simulink model "GolfSwing"  (R2024b)
settings: Solver=VariableStepAuto  StartTime=0.0  StopTime=StopTime  MaxStep=0.001  RelTol=1e-3
PreLoadFcn:
  | cd(matlabdrive);
  | cd '2DModel';
PostLoadFcn:
  | %run SCRIPT_mdlWksGenerate.m;
  | mdlWks=get_param('GolfSwing','ModelWorkspace');
  | mdlWks.DataSource = 'MAT-File';
  | mdlWks.FileName = 'ModelInputs.mat';
  | mdlWks.reload;
model workspace: external: MAT-File ModelInputs.mat (data not in the file)
undefined symbols (not defined in the file or in its folder): GlobalGain, HipConstant, HipDampening, HipTimeGain, KillDampFinalValue, KillDampInitialValue, KillswitchFinalValue, KillswitchInitialValue, KillswitchStepTime, LElbowConstant, LElbowDampening, LElbowTimeGain, LScapConstant, LScapDampening, LScapPositionGain, LScapTimeGain, LShoulderConstant, LShoulderDampening, LShoulderTimeGain, LWristConstant, LWristDampening, LWristTimeGain, RElbowConstant, RElbowDampening, RElbowTimeGain, RScapConstant, RScapDampening, RScapPositionGain, RScapTimeGain, RShoulderConstant, RShoulderDampening, RShoulderTimeGain, RWristConstant, RWristDampening, RWristTimeGain, TorsoConstant, TorsoDampening, TorsoPositionGain, TorsoTimeGain, WristGain, X, Y, Z
libraries: nesl_utility x207, sm_lib x106, matrix_library x11, simulink_extras x2, simulink x1
(part 6 of 6)

== system GolfSwing/Club/RWGlobal ==
  Add : Sum  Inputs=+++
  Math Function : Math  Operator=square
  Math Function1 : Math  Operator=square
  Math Function2 : Math  Operator=square
  Mux : Mux  Inputs=3
  Mux1 : Mux  Inputs=3
  RWAV : nesl_utility/PS-Simulink Converter  PhysicalDomain=network_engine_domain  SubClassName=ps_output  LeftPortType=input  RightPortType=output  PseudoPeriodic=off  Frequencies=[]  VectorFormat=1-D array  Unit=inherit  AffineConversion=off
  RWvx : nesl_utility/PS-Simulink Converter  PhysicalDomain=network_engine_domain  SubClassName=ps_output  LeftPortType=input  RightPortType=output  PseudoPeriodic=off  Frequencies=[]  VectorFormat=1-D array  Unit=inherit  AffineConversion=off
  RWvy : nesl_utility/PS-Simulink Converter  PhysicalDomain=network_engine_domain  SubClassName=ps_output  LeftPortType=input  RightPortType=output  PseudoPeriodic=off  Frequencies=[]  VectorFormat=1-D array  Unit=inherit  AffineConversion=off
  RWvz : nesl_utility/PS-Simulink Converter  PhysicalDomain=network_engine_domain  SubClassName=ps_output  LeftPortType=input  RightPortType=output  PseudoPeriodic=off  Frequencies=[]  VectorFormat=1-D array  Unit=inherit  AffineConversion=off
  RWx : nesl_utility/PS-Simulink Converter  PhysicalDomain=network_engine_domain  SubClassName=ps_output  LeftPortType=input  RightPortType=output  PseudoPeriodic=off  Frequencies=[]  VectorFormat=1-D array  Unit=inherit  AffineConversion=off
  RWy : nesl_utility/PS-Simulink Converter  PhysicalDomain=network_engine_domain  SubClassName=ps_output  LeftPortType=input  RightPortType=output  PseudoPeriodic=off  Frequencies=[]  VectorFormat=1-D array  Unit=inherit  AffineConversion=off
  RWz : nesl_utility/PS-Simulink Converter  PhysicalDomain=network_engine_domain  SubClassName=ps_output  LeftPortType=input  RightPortType=output  PseudoPeriodic=off  Frequencies=[]  VectorFormat=1-D array  Unit=inherit  AffineConversion=off
  RightHandPathUnitVector : Mux  Inputs=3
  RightHandSpeed : Sqrt
  Transform Sensor : sm_lib/Frames and Transforms/Transform Sensor  MeasurementFrame=World  RotationSequence=XYX  SenseAngle=off  SenseAxis=off  SenseQ=off  SenseR=off  SenseRotationSequence=off  SenseOmegaX=off  SenseOmegaY=off  SenseOmegaZ=off  SenseOmega=on  SenseQDot=off  SenseRDot=off  SenseRotationSequenceDot=off  SenseAlphaX=off  SenseAlphaY=off  SenseAlphaZ=off  SenseAlpha=off  SenseQDDot=off  SenseRDDot=off  SenseX=on  SenseY=on  SenseZ=on  SenseXYZ=off  SenseRad=off  SenseAzim=off  SenseDist=off  SenseInc=off  SenseXDot=on  SenseYDot=on  SenseZDot=on  SenseXYZDot=off  SenseRadDot=off  SenseAzimDot=off  SenseDistDot=off  SenseIncDot=off  SenseXDDot=off  SenseYDDot=off  SenseZDDot=off  SenseXYZDDot=off  SenseRadDDot=off  SenseAzimDDot=off  SenseDistDDot=off  SenseIncDDot=off
  UnitVectorX : Product  Inputs=*/
  UnitVectorY : Product  Inputs=*/
  UnitVectorZ : Product  Inputs=*/
  Conn1 : PMIOPort  Side=Right
  Conn2 : PMIOPort  Port=2  Side=Left
  RightHandPathVector : Outport
  RightHandPosition : Outport  Port=2
  RHVelocity : Outport  Port=3
  RightWristGlobalAV : Outport  Port=4
  wires:
  RightHandSpeed/1 -> UnitVectorZ/2, UnitVectorY/2, UnitVectorX/2  "RightHandSpeed"
  Math Function/1 -> Add/1
  Add/1 -> RightHandSpeed/1
  Math Function2/1 -> Add/3
  Math Function1/1 -> Add/2
  UnitVectorX/1 -> RightHandPathUnitVector/1
  RightHandPathUnitVector/1 -> RightHandPathVector/1  "RightHandPathVector"
  UnitVectorZ/1 -> RightHandPathUnitVector/3
  UnitVectorY/1 -> RightHandPathUnitVector/2
  RWy/1 -> Mux/2  "RWy"
  RWz/1 -> Mux/3  "RWz"
  Mux/1 -> RightHandPosition/1  "RightHandPosition"
  RWx/1 -> Mux/1  "RWx"
  RWvz/1 -> Math Function2/1, Mux1/3, UnitVectorZ/1  "RWvz"
  RWvy/1 -> UnitVectorY/1, Math Function1/1, Mux1/2  "RWvy"
  Mux1/1 -> RHVelocity/1  "RightHandVelocity"
  RWvx/1 -> UnitVectorX/1, Mux1/1, Math Function/1  "RWvx"
  RWAV/1 -> RightWristGlobalAV/1  "RightWristGlobalAV"
  connections:
  Transform Sensor/LConn1 -- Conn2/RConn1
  Transform Sensor/RConn1 -- Conn1/RConn1
  RWx/LConn1 -- Transform Sensor/RConn3
  RWy/LConn1 -- Transform Sensor/RConn4
  RWz/LConn1 -- Transform Sensor/RConn5
  RWvx/LConn1 -- Transform Sensor/RConn6
  RWvy/LConn1 -- Transform Sensor/RConn7
  RWvz/LConn1 -- Transform Sensor/RConn8
  RWAV/LConn1 -- Transform Sensor/RConn2

== system GolfSwing/Club/Rigid Shaft ==
  Rigid Shaft : sm_lib/Body Elements/Cylindrical Solid  CylinderRadius=0.01  CylinderRadiusUnits=m  CylinderLength=1  CylinderLengthUnits=m  ExportEntireGeometry=off  InertiaType=CalculateFromGeometry  BasedOnType=Mass  Density=500  DensityUnits=kg/m^3  Mass=0.0802566  MassUnits=kg  CenterOfMass=[0 0 0]  CenterOfMassUnits=m  MomentsOfInertia=[1 1 1]  MomentsOfInertiaUnits=kg*m^2  ProductsOfInertia=[0 0 0]  ProductsOfInertiaUnits=kg*m^2  GraphicType=FromGeometry  MarkerShape=Sphere  MarkerSize=10  GraphicVisPropType=SimpleVisualProperties  GraphicDiffuseColor=[0.5 0.5 0.5]  GraphicOpacity=1.0  GraphicSpecularColor=[0.5 0.5 0.5 1.0]  GraphicAmbientColor=[0.15 0.15 0.15 1.0]  GraphicEmissiveColor=[0.0 0.0 0.0 1.0]  GraphicShininess=75  DoExposeReferenceFrame=off  SerializedFrames=<Frames><Frame><Id>Frame1</Id><Value><Name>RHGripTOS</Name><Origin><Source>GeometricFeature</Source><FeatureName>top curve</FeatureName></Origin><PrimaryAxis><DefinedDirection>-X</DefinedDirection><Source>ReferenceFrame</Source><SourceDirection>+Z</SourceDirection><FeatureName></FeatureName></PrimaryAxis><SecondaryAxis><DefinedDirection>+Y</DefinedDirection><Source>ReferenceFrame</Source><SourceDirection>+X</SourceDirection><FeatureName></FeatureName></SecondaryAxis></Value></Frame><Frame><Id>Frame2</Id><Value><Name>ShaftS1</Name><Origin><Source>GeometricFeature</Source><FeatureName>bottom curve</FeatureName></Origin><PrimaryAxis><DefinedDirection>-X</DefinedDirection><Source>ReferenceFrame</Source><SourceDirection>+Z</SourceDirection><FeatureName></FeatureName></PrimaryAxis><SecondaryAxis><DefinedDirection>+Y</DefinedDirection><Source>ReferenceFrame</Source><SourceDirection>+X</SourceDirection><FeatureName></FeatureName></SecondaryAxis></Value></Frame></Frames>
  RH : PMIOPort  Side=Right
  Clubhead : PMIOPort  Port=2  Side=Right
  connections:
  RH/RConn1 -- Rigid Shaft/LConn1
  Clubhead/RConn1 -- Rigid Shaft/RConn1

== system GolfSwing/Club/Zero Mass Reference Shaft ==
  CHSCalculation : Subsystem  Commented=on
  CHvx : nesl_utility/PS-Simulink Converter  Commented=on  PhysicalDomain=network_engine_domain  SubClassName=ps_output  LeftPortType=input  RightPortType=output  PseudoPeriodic=off  Frequencies=[]  VectorFormat=1-D array  Unit=inherit  AffineConversion=off
  CHvy : nesl_utility/PS-Simulink Converter  Commented=on  PhysicalDomain=network_engine_domain  SubClassName=ps_output  LeftPortType=input  RightPortType=output  PseudoPeriodic=off  Frequencies=[]  VectorFormat=1-D array  Unit=inherit  AffineConversion=off
  CHvz : nesl_utility/PS-Simulink Converter  Commented=on  PhysicalDomain=network_engine_domain  SubClassName=ps_output  LeftPortType=input  RightPortType=output  PseudoPeriodic=off  Frequencies=[]  VectorFormat=1-D array  Unit=inherit  AffineConversion=off
  CHx : nesl_utility/PS-Simulink Converter  Commented=on  PhysicalDomain=network_engine_domain  SubClassName=ps_output  LeftPortType=input  RightPortType=output  PseudoPeriodic=off  Frequencies=[]  VectorFormat=1-D array  Unit=inherit  AffineConversion=off
  CHy : nesl_utility/PS-Simulink Converter  Commented=on  PhysicalDomain=network_engine_domain  SubClassName=ps_output  LeftPortType=input  RightPortType=output  PseudoPeriodic=off  Frequencies=[]  VectorFormat=1-D array  Unit=inherit  AffineConversion=off
  CHz : nesl_utility/PS-Simulink Converter  Commented=on  PhysicalDomain=network_engine_domain  SubClassName=ps_output  LeftPortType=input  RightPortType=output  PseudoPeriodic=off  Frequencies=[]  VectorFormat=1-D array  Unit=inherit  AffineConversion=off
  ClubheadPathUnitVector : Mux  Commented=on  Inputs=3
  ShaftPhysicalConfig : Subsystem
  Transform Sensor : sm_lib/Frames and Transforms/Transform Sensor  Commented=on  MeasurementFrame=World  RotationSequence=XYX  SenseAngle=off  SenseAxis=off  SenseQ=off  SenseR=off  SenseRotationSequence=off  SenseOmegaX=off  SenseOmegaY=off  SenseOmegaZ=off  SenseOmega=off  SenseQDot=off  SenseRDot=off  SenseRotationSequenceDot=off  SenseAlphaX=off  SenseAlphaY=off  SenseAlphaZ=off  SenseAlpha=off  SenseQDDot=off  SenseRDDot=off  SenseX=on  SenseY=on  SenseZ=on  SenseXYZ=off  SenseRad=off  SenseAzim=off  SenseDist=off  SenseInc=off  SenseXDot=on  SenseYDot=on  SenseZDot=on  SenseXYZDot=off  SenseRadDot=off  SenseAzimDot=off  SenseDistDot=off  SenseIncDot=off  SenseXDDot=off  SenseYDDot=off  SenseZDDot=off  SenseXYZDDot=off  SenseRadDDot=off  SenseAzimDDot=off  SenseDistDDot=off  SenseIncDDot=off
  UnitVectorX : Product  Commented=on  Inputs=*/
  UnitVectorY : Product  Commented=on  Inputs=*/
  UnitVectorZ : Product  Commented=on  Inputs=*/
  RH : PMIOPort  Side=Right
  ConnGlobal : PMIOPort  Port=2  Side=Right
  wires:
  CHvz/1 -> CHSCalculation/3(In1), UnitVectorZ/1
  CHvy/1 -> CHSCalculation/2(In3), UnitVectorY/1
  UnitVectorY/1 -> ClubheadPathUnitVector/2
  UnitVectorZ/1 -> ClubheadPathUnitVector/3
  CHSCalculation/1(Out1) -> UnitVectorY/2, UnitVectorZ/2, UnitVectorX/2  "GhostCHS"
  UnitVectorX/1 -> ClubheadPathUnitVector/1
  CHvx/1 -> CHSCalculation/1(In2), UnitVectorX/1
  connections:
  ShaftPhysicalConfig/RConn1 -- RH/RConn1
  ConnGlobal/RConn1 -- Transform Sensor/LConn1
  ShaftPhysicalConfig/RConn2 -- Transform Sensor/RConn1
  CHy/LConn1 -- Transform Sensor/RConn3
  CHvy/LConn1 -- Transform Sensor/RConn6
  CHx/LConn1 -- Transform Sensor/RConn2
  CHz/LConn1 -- Transform Sensor/RConn4
  CHvz/LConn1 -- Transform Sensor/RConn7
  CHvx/LConn1 -- Transform Sensor/RConn5

== system GolfSwing/Right Wrist Joint/RightWristRelease ==
  note: To operate the right wrist release you need to set the right wrist joint configuration to "Provided by input" and then put this step function on the input and give it a release time and then the right hand will let go at that point in time.
  RIght Wrist Release : Step  Commented=on  After=-1  SampleTime=0
  Simulink-PS Converter : nesl_utility/Simulink-PS Converter  Commented=on  PhysicalDomain=network_engine_domain  SubClassName=ps_input  LeftPortType=input  RightPortType=output  PseudoPeriodic=off  Frequencies=[]  NoiseDistribution=none  NoiseParameters=[]  Unit=1  AffineConversion=off  FilteringAndDerivatives=provide  SimscapeFilterOrder=1  InputFilterTimeConstant=0.001  UdotUserProvided=0
  output : PMIOPort  Side=Right
  wires:
  RIght Wrist Release/1 -> Simulink-PS Converter/1
  connections:
  Simulink-PS Converter/RConn1 -- output/RConn1

== system GolfSwing/Club/CHGlobal/AoA Calculation ==
  Vx : Inport
  Vy : Inport  Port=2
  Vz : Inport  Port=3
  Add : Sum
  AoA : simulink_extras/Transformations/Radians to Degrees
  Divide : Product  Inputs=*/
  Run : Sqrt
  Square : Math  Operator=square
  Square1 : Math  Operator=square
  atan : Trigonometry  Operator=atan
  wires:
  Vy/1 -> Square1/1
  Square/1 -> Add/1
  Run/1 -> Divide/2
  Square1/1 -> Add/2
  Vz/1 -> Divide/1
  Divide/1 -> atan/1
  Add/1 -> Run/1
  Vx/1 -> Square/1
  atan/1 -> AoA/1

== system GolfSwing/Club/CHGlobal/CHS (m//s) ==
  In1 : Inport
  In2 : Inport  Port=2
  In3 : Inport  Port=3
  Add : Sum  Inputs=+++
  Math Function : Math  Operator=square
  Math Function1 : Math  Operator=square
  Math Function2 : Math  Operator=square
  Sqrt : Sqrt
  ClubPathUV1 : Outport
  wires:
  Math Function2/1 -> Add/3
  In1/1 -> Math Function/1
  In2/1 -> Math Function1/1
  Math Function/1 -> Add/1
  Add/1 -> Sqrt/1
  In3/1 -> Math Function2/1
  Sqrt/1 -> ClubPathUV1/1
  Math Function1/1 -> Add/2

== system GolfSwing/Club/CHGlobal/Filtering Block ==
  CHS (mph) : Inport
  MATLAB Function : MATLAB Function  Commented=on  TreatAsAtomicUnit=on
  wires:
  CHS (mph)/1 -> MATLAB Function/1(u)

== system GolfSwing/Club/CHGlobal/Path Calculation ==
  Vy : Inport
  Vx : Inport  Port=2
  Constant : Constant  Value=-1
  Divide : Product  Inputs=*/
  Path : simulink_extras/Transformations/Radians to Degrees
  PathCalc : Trigonometry  Operator=atan
  Product : Product
  wires:
  Vy/1 -> Divide/1
  Divide/1 -> PathCalc/1
  PathCalc/1 -> Product/1
  Vx/1 -> Divide/2
  Product/1 -> Path/1
  Constant/1 -> Product/2

== system GolfSwing/Club/Zero Mass Reference Shaft/CHSCalculation ==
  In2 : Inport
  In3 : Inport  Port=2
  In1 : Inport  Port=3
  Add : Sum  Inputs=+++
  Math Function : Math  Operator=square
  Math Function1 : Math  Operator=square
  Math Function2 : Math  Operator=square
  Sqrt : Sqrt
  Out1 : Outport
  wires:
  Math Function2/1 -> Add/3
  In1/1 -> Math Function/1
  In2/1 -> Math Function1/1
  Math Function/1 -> Add/1
  Add/1 -> Sqrt/1
  In3/1 -> Math Function2/1
  Sqrt/1 -> Out1/1
  Math Function1/1 -> Add/2

== system GolfSwing/Club/Zero Mass Reference Shaft/ShaftPhysicalConfig ==
  GhostShaft : sm_lib/Body Elements/Cylindrical Solid  CylinderRadius=0.01  CylinderRadiusUnits=m  CylinderLength=1  CylinderLengthUnits=m  ExportEntireGeometry=off  InertiaType=CalculateFromGeometry  BasedOnType=Mass  Density=500  DensityUnits=kg/m^3  Mass=0  MassUnits=kg  CenterOfMass=[0 0 0]  CenterOfMassUnits=m  MomentsOfInertia=[1 1 1]  MomentsOfInertiaUnits=kg*m^2  ProductsOfInertia=[0 0 0]  ProductsOfInertiaUnits=kg*m^2  GraphicType=FromGeometry  MarkerShape=Sphere  MarkerSize=10  GraphicVisPropType=SimpleVisualProperties  GraphicDiffuseColor=[0.2 0.2 1.0]  GraphicOpacity=1.0  GraphicSpecularColor=[0.5 0.5 0.5 1.0]  GraphicAmbientColor=[0.15 0.15 0.15 1.0]  GraphicEmissiveColor=[0.0 0.0 0.0 1.0]  GraphicShininess=75  DoExposeReferenceFrame=off  SerializedFrames=<Frames><Frame><Id>Frame1</Id><Value><Name>RHGripTOS</Name><Origin><Source>GeometricFeature</Source><FeatureName>top curve</FeatureName></Origin><PrimaryAxis><DefinedDirection>-X</DefinedDirection><Source>ReferenceFrame</Source><SourceDirection>+Z</SourceDirection><FeatureName></FeatureName></PrimaryAxis><SecondaryAxis><DefinedDirection>+Y</DefinedDirection><Source>ReferenceFrame</Source><SourceDirection>+X</SourceDirection><FeatureName></FeatureName></SecondaryAxis></Value></Frame><Frame><Id>Frame2</Id><Value><Name>GhostClubhead</Name><Origin><Source>GeometricFeature</Source><FeatureName>bottom curve</FeatureName></Origin><PrimaryAxis><DefinedDirection>+Z</DefinedDirection><Source>ReferenceFrame</Source><SourceDirection>+Z</SourceDirection><FeatureName></FeatureName></PrimaryAxis><SecondaryAxis><DefinedDirection>+X</DefinedDirection><Source>ReferenceFrame</Source><SourceDirection>+X</SourceDirection><FeatureName></FeatureName></SecondaryAxis></Value></Frame></Frames>
  PS-Simulink Converter14 : nesl_utility/PS-Simulink Converter  PhysicalDomain=network_engine_domain  SubClassName=ps_output  LeftPortType=input  RightPortType=output  PseudoPeriodic=off  Frequencies=[]  VectorFormat=inherit  Unit=inherit  AffineConversion=off
  RH : PMIOPort  Side=Right
  RH1 : PMIOPort  Port=2  Side=Right
  connections:
  GhostShaft/LConn1 -- RH/RConn1
  RH1/RConn1 -- GhostShaft/RConn1

== matlab function GolfSwing/RJM Inputs/Left Shoulder Input Torque ==
  data: Time input; LeftShoulderTimeGain input; JointTorqueLShoulder output; LeftShoulderConstant input; LeftShoulderVelocity input; LeftShoulderDamper input; Killswitch input; GlobalGain input; KillDamp input
function JointTorqueLShoulder = fcn(Time,LeftShoulderTimeGain,LeftShoulderConstant,LeftShoulderVelocity,LeftShoulderDamper,Killswitch,GlobalGain,KillDamp)
JointTorqueLShoulder = Killswitch*GlobalGain*(LeftShoulderTimeGain*Time+LeftShoulderConstant)-GlobalGain*KillDamp*(LeftShoulderVelocity*LeftShoulderDamper);

== matlab function GolfSwing/RJM Inputs/Right Shoulder Input Torque ==
  data: Time input; RightShoulderTimeGain input; JointTorqueRShoulder output; RightShoulderConstant input; RightShoulderVelocity input; RightShoulderDamper input; Killswitch input; GlobalGain input; KillDamp input
function JointTorqueRShoulder = fcn(Time,RightShoulderTimeGain,RightShoulderConstant,RightShoulderVelocity,RightShoulderDamper,Killswitch,GlobalGain,KillDamp)
JointTorqueRShoulder = Killswitch*GlobalGain*(RightShoulderTimeGain*Time+RightShoulderConstant)-GlobalGain*KillDamp*RightShoulderVelocity*RightShoulderDamper;

== matlab function GolfSwing/RJM Inputs/Left Wrist Input Torque ==
  data: Time input; LeftWristTimeGain input; JointTorqueLWrist output; LeftWristConstant input; LeftWristVelocity input; LeftWristDamper input; Killswitch input; GlobalGain input; KillDamp input; WristGain input
function JointTorqueLWrist = fcn(Time,LeftWristTimeGain,LeftWristConstant,LeftWristVelocity,LeftWristDamper,Killswitch,GlobalGain,KillDamp,WristGain)
JointTorqueLWrist = WristGain*(Killswitch*GlobalGain*(LeftWristTimeGain*Time+LeftWristConstant)-GlobalGain*KillDamp*LeftWristVelocity*LeftWristDamper);

== matlab function GolfSwing/RJM Inputs/Right Wrist Input Torque ==
  data: Time input; RightWristTimeGain input; JointTorqueRWrist output; RightWristConstant input; RightWristVelocity input; RightWristDamper input; Killswitch input; GlobalGain input; KillDamp input; WristGain input
function JointTorqueRWrist = fcn(Time,RightWristTimeGain,RightWristConstant,RightWristVelocity,RightWristDamper,Killswitch,GlobalGain,KillDamp,WristGain)
JointTorqueRWrist = WristGain*(Killswitch*GlobalGain*(RightWristTimeGain*Time+RightWristConstant)-GlobalGain*KillDamp*RightWristVelocity*RightWristDamper);

== matlab function GolfSwing/RJM Inputs/Left Elbow Input Torque ==
  data: Time input; LeftElbowTimeGain input; JointTorqueLElbow output; LeftElbowConstant input; LeftElbowVelocity input; LeftElbowDamper input; Killswitch input; GlobalGain input; KillDamp input
function JointTorqueLElbow = fcn(Time,LeftElbowTimeGain,LeftElbowConstant,LeftElbowVelocity,LeftElbowDamper,Killswitch,GlobalGain,KillDamp)
JointTorqueLElbow = Killswitch*GlobalGain*(LeftElbowTimeGain*Time+LeftElbowConstant)-GlobalGain*KillDamp*LeftElbowVelocity*LeftElbowDamper;

== matlab function GolfSwing/RJM Inputs/Right Elbow Input Torque ==
  data: Time input; RightElbowTimeGain input; JointTorqueRElbow output; RightElbowConstant input; RightElbowVelocity input; RightElbowDamper input; Killswitch input; GlobalGain input; KillDamp input
function JointTorqueRElbow = fcn(Time,RightElbowTimeGain,RightElbowConstant,RightElbowVelocity,RightElbowDamper,Killswitch,GlobalGain,KillDamp)
JointTorqueRElbow = Killswitch*GlobalGain*(RightElbowTimeGain*Time+RightElbowConstant)-GlobalGain*KillDamp*(RightElbowVelocity*RightElbowDamper);

== matlab function GolfSwing/Club/CHGlobal/Filtering Block/MATLAB Function ==
  data: u input; y output
function y = fcn(u)
% Need to figure out how to design a filter and use the filtfilt function
% as it is a zero phase shift filter.

% function y = fcn(u)
% 
% y = filtfilt();

== matlab function GolfSwing/RJM Inputs/DeltaFunction ==
  data: Time input; WristGain input; LeftWristTimeGain input; JointTorqueDelta output; LeftWristConstant input; LeftWristVelocity input; LeftWristDamper input; Killswitch input; GlobalGain input; KillDamp input; RightWristTimeGain input; RightWristConstant input; RightWristVelocity input; RightWristDamper input; LeftElbowTimeGain input; LeftElbowConstant input; LeftElbowVelocity input; LeftElbowDamper input; RightElbowTimeGain input; RightElbowConstant input; RightElbowVelocity input; RightElbowDamper input; LeftShoulderTimeGain input; LeftShoulderConstant input; LeftShoulderVelocity input; LeftShoulderDamper input; RightShoulderTimeGain input; RightShoulderConstant input; RightShoulderVelocity input; RightShoulderDamper input
function JointTorqueDelta = fcn(Time,WristGain,LeftWristTimeGain,LeftWristConstant,LeftWristVelocity,LeftWristDamper,Killswitch,GlobalGain,KillDamp,RightWristTimeGain,RightWristConstant,RightWristVelocity,RightWristDamper,LeftElbowTimeGain,LeftElbowConstant,LeftElbowVelocity,LeftElbowDamper,RightElbowTimeGain,RightElbowConstant,RightElbowVelocity,RightElbowDamper,LeftShoulderTimeGain,LeftShoulderConstant,LeftShoulderVelocity,LeftShoulderDamper,RightShoulderTimeGain,RightShoulderConstant,RightShoulderVelocity,RightShoulderDamper)

% Turn off delta function:
JointTorqueDelta = 0;

% In order to make left wrist torque equal to zero, the delta needs to be
% set to the following function:
% JointTorqueDelta = -(WristGain*(Killswitch*GlobalGain*(LeftWristTimeGain*Time+LeftWristConstant)-GlobalGain*KillDamp*LeftWristVelocity*LeftWristDamper));

% In order to make right wrist torque equal to zero, the delta needs to be
% set to the following function:
% JointTorqueDelta = WristGain*(Killswitch*GlobalGain*(RightWristTimeGain*Time+RightWristConstant)-GlobalGain*KillDamp*RightWristVelocity*RightWristDamper);

% In order to make left elbow torque equal to zero, the delta needs to be
% set to the following function:
% JointTorqueDelta = -(Killswitch*GlobalGain*(LeftElbowTimeGain*Time+LeftElbowConstant)-GlobalGain*KillDamp*LeftElbowVelocity*LeftElbowDamper);

% In order to make right elbow torque equal to zero, the delta needs to be
% set to the following function:
% JointTorqueDelta = (Killswitch*GlobalGain*(RightElbowTimeGain*Time+RightElbowConstant)-GlobalGain*KillDamp*(RightElbowVelocity*RightElbowDamper));

% In order to make left shoulder torque equal to zero, the delta needs to be
% set to the following function:
% JointTorqueDelta = -(Killswitch*GlobalGain*(LeftShoulderTimeGain*Time+LeftShoulderConstant)-GlobalGain*KillDamp*(LeftShoulderVelocity*LeftShoulderDamper));

% In order to make right shoulder torque equal to zero, the delta needs to be
% set to the following function:
% JointTorqueDelta = (Killswitch*GlobalGain*(RightShoulderTimeGain*Time+RightShoulderConstant)-GlobalGain*KillDamp*RightShoulderVelocity*RightShoulderDamper);

% To split the wrist torque equally between the left and right wrist use
% the following fomula.
% JointTorqueDelta=-(WristGain*(Killswitch*GlobalGain*(LeftWristTimeGain*Time+LeftWristConstant)-GlobalGain*KillDamp*LeftWristVelocity*LeftWristDamper))+((WristGain*(Killswitch*GlobalGain*(LeftWristTimeGain*Time+LeftWristConstant)-GlobalGain*KillDamp*LeftWristVelocity*LeftWristDamper))+WristGain*(Killswitch*GlobalGain*(RightWristTimeGain*Time+RightWristConstant)-GlobalGain*KillDamp*RightWristVelocity*RightWristDamper))/2;

== matlab function GolfSwing/MATLAB Function ==
  data: LateralConstant input; LateralForce output; LateralTimeGain input; Time input
function LateralForce = fcn(LateralConstant,LateralTimeGain,Time)

LateralForce = LateralConstant-Time*LateralTimeGain;

== matlab function GolfSwing/Club/Impact Model/Golf Ball Reaction Force ==
  data: u input; FImpact output
function FImpact = fcn(u)

FImpact=-u*1.5*.44704*.0459/.0005;
%Impact Time = 0.0005 s
%Golf Ball Mass = 0.0459 g
%MPH to m/s conversion = 0.44704 m/s / MPH
%Smash Factor = 1.5

== matlab function GolfSwing/Club/Clubhead Air Resistance Calculator/Drag Function ==
  data: u input; FDrag output
function FDrag = fcn(u)

FDrag = -1/2*1.225*3.1415927*(2.5/39)^2*0.47*u^2;
%Shape Factor = 0.47
%Air Density = 1.225 kg/m3
%CH Radius = 2.5"
%Fd=-1/2*Density*ShapeFactor*CSA*v^2

== matlab function GolfSwing/RJM Inputs/Hip Input Torque ==
  data: Time input; HipTimeGain input; JointTorqueHips output; HipConstant input; HipVelocity input; HipDamper input; Killswitch input; GlobalGain input; KillDamp input
% Time factor has been changed to depend on t^2 rather than t to get more
% drop off with time.

function JointTorqueHips = fcn(Time,HipTimeGain,HipConstant,HipVelocity,HipDamper,Killswitch,GlobalGain,KillDamp)
JointTorqueHips=Killswitch*GlobalGain*(HipTimeGain*Time+HipConstant)-GlobalGain*KillDamp*HipVelocity*HipDamper;

== matlab function GolfSwing/RJM Inputs/Torso Input Torque ==
  data: Time input; TorsoTimeGain input; JointTorqueTorso output; TorsoConstant input; TorsoVelocity input; TorsoDamper input; TorsoPosition input; TorsoPositionGain input; Killswitch input; GlobalGain input; KillDamp input
function JointTorqueTorso = fcn(Time,TorsoTimeGain,TorsoConstant,TorsoVelocity,TorsoDamper,TorsoPosition,TorsoPositionGain,Killswitch,GlobalGain,KillDamp)
JointTorqueTorso = Killswitch*GlobalGain*(TorsoTimeGain*Time+TorsoConstant-TorsoPositionGain*TorsoPosition)-GlobalGain*KillDamp*TorsoVelocity*TorsoDamper;

== matlab function GolfSwing/RJM Inputs/LScap Input Torque ==
  data: Time input; LScapTimeGain input; JointTorqueLScap output; LScapConstant input; LScapVelocity input; LScapDamper input; LScapPosition input; LScapPositionGain input; Killswitch input; GlobalGain input; KillDamp input
function JointTorqueLScap = fcn(Time,LScapTimeGain,LScapConstant,LScapVelocity,LScapDamper,LScapPosition,LScapPositionGain,Killswitch,GlobalGain,KillDamp)

% Scapula Excluded Scapula Damper Excluded in Killswitch:
JointTorqueLScap=GlobalGain*(LScapTimeGain*Time+LScapConstant-LScapPositionGain*LScapPosition)-GlobalGain*LScapVelocity*LScapDamper;

% Scapula Included Damper Included in Killswitch
%JointTorqueLScap=GlobalGain*Killswitch*(LScapTimeGain*Time+LScapConstant-LScapPositionGain*LScapPosition)-GlobalGain*KillDamp*LScapVelocity*LScapDamper;

% Scapula Excluded Damper Included in Killswitch
% JointTorqueRScap=GlobalGain*(LScapTimeGain*Time+LScapConstant-LScapPositionGain*LScapPosition)-GlobalGain*KillDamp*LScapVelocity*LScapDamper;

== matlab function GolfSwing/RJM Inputs/RScap Input Torque ==
  data: Time input; RScapTimeGain input; JointTorqueRScap output; RScapConstant input; RScapVelocity input; RScapDamper input; RScapPosition input; RScapPositionGain input; Killswitch input; GlobalGain input; KillDamp input
function JointTorqueRScap = fcn(Time,RScapTimeGain,RScapConstant,RScapVelocity,RScapDamper,RScapPosition,RScapPositionGain,Killswitch,GlobalGain,KillDamp)

% Scapula Excluded in Killswitch Scapula Damper Excluded in Killswitch
JointTorqueRScap = GlobalGain*(RScapTimeGain*Time+RScapConstant-RScapPositionGain*RScapPosition)-GlobalGain*RScapVelocity*RScapDamper;

% Scapula Included in Killswitch, Damper Included in Killswitch
%JointTorqueRScap = GlobalGain*Killswitch*(RScapTimeGain*Time+RScapConstant-RScapPositionGain*RScapPosition)-GlobalGain*KillDamp*RScapVelocity*RScapDamper;

% Scapula Excluded in Killswitch, Damper Included in Killswitch
% JointTorqueRScap = GlobalGain*(RScapTimeGain*Time+RScapConstant-RScapPositionGain*RScapPosition)-GlobalGain*KillDamp*RScapVelocity*RScapDamper;
